simulink model "three_phase_2_level_CMI_PWM"  (R2023b)
settings: Solver=ode23tb  StartTime=0.0  StopTime=60e-3  MaxStep=1e-6  RelTol=1e-3
libraries: spsIGBTDiodeLib x6, spsPWMGenerator2LevelLib x3, spsCurrentMeasurementLib x3, spsSeriesRLCBranchLib x3, spsVoltageMeasurementLib x3, spsDCVoltageSourceLib x1, spsGroundLib x1, spspowerguiLib x1
settings Model: Creator=divya  LastModifiedBy=divya
settings DataIOCC: ReturnWorkspaceOutputs=off

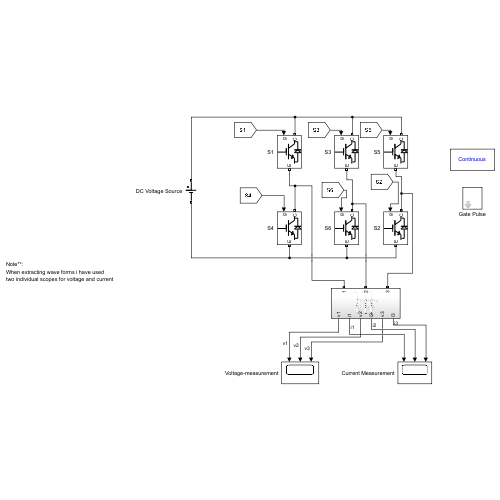
[thumbnail: Simulink's stored preview of the top-level diagram]
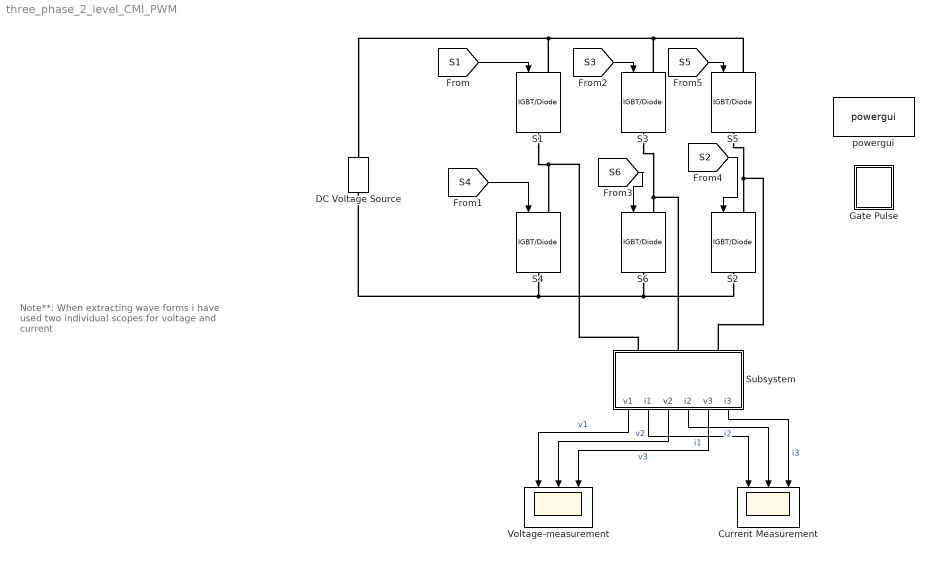
== system three_phase_2_level_CMI_PWM ==
  note: Note**:
      | When extracting wave forms i have used
      | two individual scopes for voltage and current
  Current Measurement : Scope  NumInputPorts=3
  DC Voltage Source : spsDCVoltageSourceLib/DC Voltage Source  Amplitude=100  Measurements=None
  Gate Pulse : Subsystem  mask{ma=1.15}
      mask prompts: ma "modulation index"
  S{1..6} (6 alike) : spsIGBTDiodeLib/IGBT//Diode  Ron=1e-3  Rs=1e5  Cs=inf  Measurements=off
  Subsystem : Subsystem
  Voltage-measurement : Scope  NumInputPorts=3
  powergui : spspowerguiLib/powergui  Priority=1  SimulationMode=Continuous  SampleTime=50e-6  frequency=60  Iterations=50  frequencyindice=0  Pbase=100e6  ErrMax=1e-4  UnitsV=kV  UnitsW=MW  buscounter=0  FunctionMessages=off  echomessages=off  EnableUseOfTLC=off  CurrentSourceSwitches=off  DisableSnubberDevices=off  DisableRonSwitches=off  DisableVfSwitches=off  DisplayEquations=off  AutomaticDiscreteSolvers=off  SolverType=Tustin/Backward Euler (TBE)  Interpol=off  ExternalGateDelay=off  methode=off  Ts=100  x0status=blocks  SPID=on  SwTol=0  HookPort=off  NonlinearTolerance=1e-4  nMaxIteration=100  ContinueOnMaxIteration=off  RestoreLinks=warning  ResistiveCurrentMeasurement=off  Frange=[0:2:500]  Ylog=off  Xlog=on  ShowGrid=off  save=off  variable=ZData  structure=0  ZoomFFT=off  StartTime=0.0  cycles=1  DisplayStyle=1  fundamental=60  FreqAxis=off  MaxFrequency=1000  frequencyindicesteady=1  RmsSteady=1  display=off
  wires:
  Subsystem/1(v1) -> Voltage-measurement/1  "v1"
  Subsystem/2(i1) -> Current Measurement/1  "i1"
  Subsystem/3(v2) -> Voltage-measurement/2  "v2"
  Subsystem/4(i2) -> Current Measurement/2  "i2"
  Subsystem/5(v3) -> Voltage-measurement/3  "v3"
  Subsystem/6(i3) -> Current Measurement/3  "i3"
  [S1] -> S1/1
  [S4] -> S4/1
  [S3] -> S3/1
  [S6] -> S6/1
  [S2] -> S2/1
  [S5] -> S5/1
  connections:
  S1/RConn1 -- Subsystem/LConn1 -- S4/LConn1
  S3/RConn1 -- Subsystem/LConn2 -- S6/LConn1
  S5/RConn1 -- Subsystem/LConn3 -- S2/LConn1
  S5/LConn1 -- S3/LConn1 -- S1/LConn1 -- DC Voltage Source/RConn1
  S2/RConn1 -- S6/RConn1 -- S4/RConn1 -- DC Voltage Source/LConn1

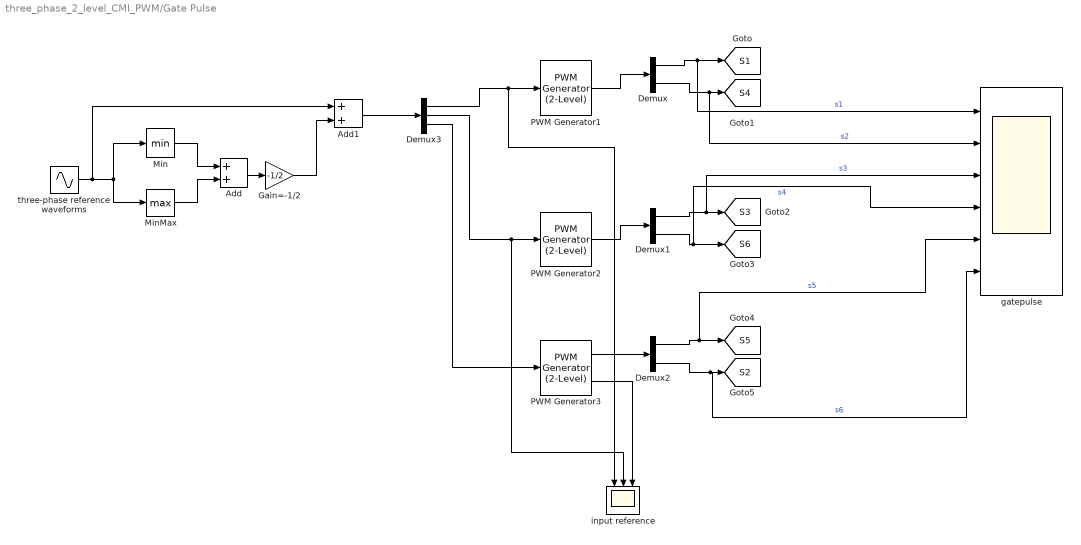
== system three_phase_2_level_CMI_PWM/Gate Pulse ==
  Add : Sum
  Add1 : Sum
  Demux : Demux  Outputs=2
  Demux1 : Demux  Outputs=2
  Demux2 : Demux  Outputs=2
  Demux3 : Demux  Outputs=3
  Gain=-1/2 : Gain  Gain=-1/2
  Min : MinMax
  MinMax : MinMax  Function=max
  PWM Generator1 : spsPWMGenerator2LevelLib/PWM Generator (2-Level)  ModulatorType=Single-phase half-bridge (2 pulses)  ModulatorMode=Unsynchronized  Fc=45*50  Pc=90  nF=27  MinMax="[ -1  1 ]"  SamplingTechnique=Natural  ModulatingSignals=off  m=0.8  Freq=60  Phase=0  Ts=0  ShowCarrierOutport=off
  PWM Generator2 : spsPWMGenerator2LevelLib/PWM Generator (2-Level)  ModulatorType=Single-phase half-bridge (2 pulses)  ModulatorMode=Unsynchronized  Fc=45*50  Pc=90  nF=27  MinMax="[ -1  1 ]"  SamplingTechnique=Natural  ModulatingSignals=off  m=0.8  Freq=60  Phase=0  Ts=0  ShowCarrierOutport=off
  PWM Generator3 : spsPWMGenerator2LevelLib/PWM Generator (2-Level)  ModulatorType=Single-phase half-bridge (2 pulses)  ModulatorMode=Unsynchronized  Fc=45*50  Pc=90  nF=27  MinMax="[ -1  1 ]"  SamplingTechnique=Natural  ModulatingSignals=off  m=0.8  Freq=60  Phase=0  Ts=0  ShowCarrierOutport=on
  gatepulse : Scope  NumInputPorts=6
  input reference : Scope  NumInputPorts=3
  three-phase reference waveforms : Sin  Amplitude=ma  Frequency=2*pi*50  Phase=[0 -2*pi/3 2*pi/3]  SampleTime=0
  tag scope: S1=global, S2=global, S3=global, S4=global, S5=global, S6=global
  wires:
  Demux2/1 -> gatepulse/5, [S5]  "s5"
  Demux2/2 -> gatepulse/6, [S2]  "s6"
  PWM Generator3/1 -> Demux2/1
  Demux/1 -> gatepulse/1, [S1]  "s1"
  PWM Generator2/1 -> Demux1/1
  Demux1/1 -> gatepulse/3, [S3]  "s3"
  Demux1/2 -> gatepulse/4, [S6]  "s4"
  Demux/2 -> gatepulse/2, [S4]  "s2"
  PWM Generator1/1 -> Demux/1
  three-phase reference waveforms/1 -> Add1/1, MinMax/1, Min/1
  Min/1 -> Add/1
  MinMax/1 -> Add/2
  Add/1 -> Gain=-1/2/1
  Gain=-1/2/1 -> Add1/2
  Add1/1 -> Demux3/1
  Demux3/1 -> input reference/1, PWM Generator1/1
  Demux3/2 -> input reference/2, PWM Generator2/1
  Demux3/3 -> PWM Generator3/1
  PWM Generator3/2 -> input reference/3

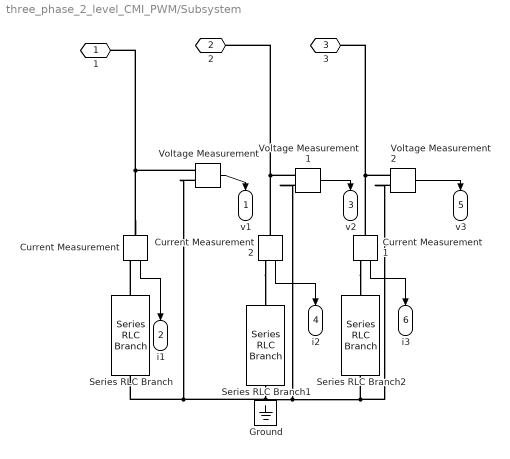
== system three_phase_2_level_CMI_PWM/Subsystem ==
  Current Measurement : spsCurrentMeasurementLib/Current Measurement  PhasorSimulation=off  OutputType=Complex  PSBequivalent=0
  Current Measurement1 : spsCurrentMeasurementLib/Current Measurement  PhasorSimulation=off  OutputType=Complex  PSBequivalent=0
  Current Measurement2 : spsCurrentMeasurementLib/Current Measurement  PhasorSimulation=off  OutputType=Complex  PSBequivalent=0
  Ground : spsGroundLib/Ground  LConnTagsString=a
  Series RLC Branch : spsSeriesRLCBranchLib/Series RLC Branch  LConnTagsString=__new0  RConnTagsString=__new0  BranchType=RL  Resistance=10  Inductance=8e-3  SetiL0=off  InitialCurrent=0  Capacitance=1e-6  Setx0=off  InitialVoltage=0  Measurements=None
  Series RLC Branch1 : spsSeriesRLCBranchLib/Series RLC Branch  LConnTagsString=__new0  RConnTagsString=__new0  BranchType=RL  Resistance=10  Inductance=8e-3  SetiL0=off  InitialCurrent=0  Capacitance=1e-6  Setx0=off  InitialVoltage=0  Measurements=None
  Series RLC Branch2 : spsSeriesRLCBranchLib/Series RLC Branch  LConnTagsString=__new0  RConnTagsString=__new0  BranchType=RL  Resistance=10  Inductance=8e-3  SetiL0=off  InitialCurrent=0  Capacitance=1e-6  Setx0=off  InitialVoltage=0  Measurements=None
  Voltage Measurement : spsVoltageMeasurementLib/Voltage Measurement  PhasorSimulation=off  OutputType=Complex  PSBequivalent=0
  Voltage Measurement1 : spsVoltageMeasurementLib/Voltage Measurement  PhasorSimulation=off  OutputType=Complex  PSBequivalent=0
  Voltage Measurement2 : spsVoltageMeasurementLib/Voltage Measurement  PhasorSimulation=off  OutputType=Complex  PSBequivalent=0
  1 : PMIOPort  Side=Left
  2 : PMIOPort  Port=2  Side=Left
  3 : PMIOPort  Port=3  Side=Left
  v1 : Outport
  i1 : Outport  Port=2
  v2 : Outport  Port=3
  i2 : Outport  Port=4
  v3 : Outport  Port=5
  i3 : Outport  Port=6
  wires:
  Voltage Measurement/1 -> v1/1
  Current Measurement2/1 -> i2/1
  Current Measurement1/1 -> i3/1
  Voltage Measurement1/1 -> v2/1
  Voltage Measurement2/1 -> v3/1
  Current Measurement/1 -> i1/1
  connections:
  Series RLC Branch/LConn1 -- Current Measurement/RConn1
  Series RLC Branch1/RConn1 -- Voltage Measurement1/LConn2 -- Voltage Measurement2/LConn2 -- Series RLC Branch2/RConn1 -- Voltage Measurement/LConn2 -- Series RLC Branch/RConn1
  Current Measurement1/RConn1 -- Series RLC Branch2/LConn1
  Voltage Measurement/LConn1 -- Current Measurement/LConn1 -- 1/RConn1
  Voltage Measurement1/LConn1 -- Current Measurement2/LConn1 -- 2/RConn1
  Current Measurement2/RConn1 -- Series RLC Branch1/LConn1
  Voltage Measurement2/LConn1 -- Current Measurement1/LConn1 -- 3/RConn1
